simulink model "androidraspberrypisensehat"  (R2025b)
settings: Solver=FixedStepAuto  StartTime=0.0  StopTime=10.0  RelTol=1e-3
libraries: androiduilib x6, androidcommunicationlib x2
settings Model: Creator=The MathWorks, Inc.  LastModifiedBy=The MathWorks, Inc.
settings SolverCC: AlgebraicLoopSolver=TrustRegion  MaxZcPerStep=1.0
settings OptimizationCC: EnhancedBackFolding=on  PassReuseOutputArgsThreshold=0.0  MaxStackSize=64  OptimizeBlockOrder=speed  DifferentSizesBufferReuse=on  OptimizationCustomize=off
settings DebuggingCC: ParameterTunabilityLossMsg=error  UnconnectedInputMsg=warning  UnconnectedOutputMsg=warning  UnconnectedLineMsg=warning
settings HardwareCC: ProdBitPerPointer=32.0  ProdBitPerSizeT=32.0  ProdBitPerPtrDiffT=32.0  ProdLargestAtomicInteger=Long  ProdLargestAtomicFloat=Double  ProdWordSize=32.0  ProdHWDeviceType=ARM Compatible->ARM Cortex-A (32-bit)  UseEmbeddedCoderFeatures=off  UseSimulinkCoderFeatures=off
settings ModelReferenceCC: EnableRefExpFcnMdlSchedulingChecks=on
settings SFSimCC: MATLABDynamicMemAlloc=off
settings RTWCC: SystemTargetFile=ert.tlc  HardwareBoard=Android Device  TLCOptions="-aInlineSetEventsForThisBaseRateFcn=TLC_FALSE -aSuppressMultiTaskScheduler=TLC_FALSE  -aRateBasedStepFcn=0"  TemplateMakefile=ert_default_tmf  GenerateReport=on  RTWVerbose=off  Toolchain=Android SDK/NDK Tools  LaunchReport=on  GPUComputeCapability=3.5  DLArmComputeVersion=19.05  Description=Embedded Coder
settings CodeAppCC: ForceParamTrailComments=on  OperatorAnnotations=on
settings ERTTargetCC: InlinedParameterPlacement=Hierarchical  DynamicArrayContainerType=coder::array  ERTCustomFileBanners=off  SupportContinuousTime=on  SupportNonInlinedSFcns=on  RemoveResetFunc=off  ModelStepFunctionPrototypeControlCompliant=off

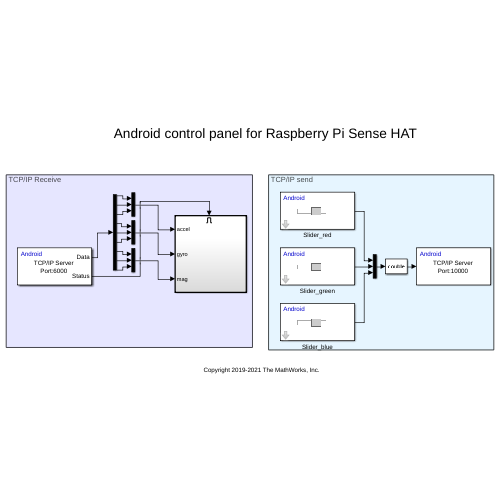
[thumbnail: Simulink's stored preview of the top-level diagram]
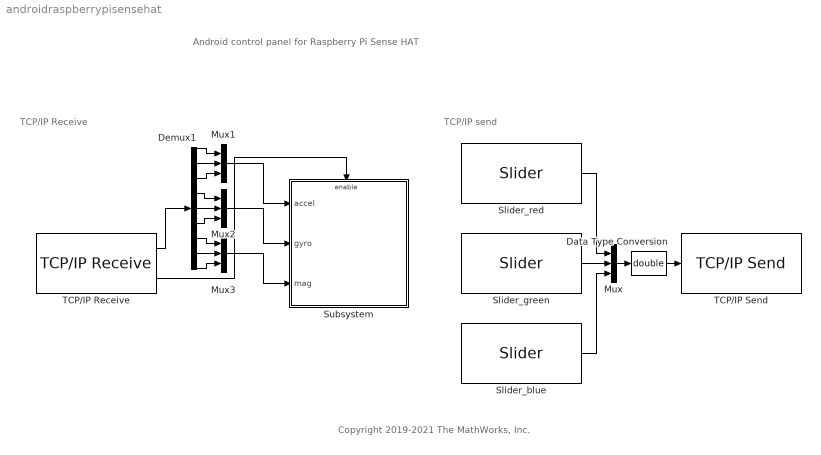
== system androidraspberrypisensehat ==
  note: Android control panel for Raspberry Pi Sense HAT
  note: TCP/IP send
  note: TCP/IP Receive
  note: Copyright 2019-2021 The MathWorks, Inc.
  Data Type Conversion : DataTypeConversion  OutDataTypeStr=double  SaturateOnIntegerOverflow=off  RndMeth=Floor
  Demux1 : Demux  Outputs=9
  Mux{,1..3} (4 alike) : Mux  Inputs=3
  Slider_blue : androiduilib/Slider  Min=1  Value=1  Max=255  Resolution=1  SliderId=androidraspberrypisensehat/Slider_blue  SampleTime=0.5  BlockPlatform=Android
  Slider_green : androiduilib/Slider  Min=1  Value=1  Max=255  Resolution=1  SliderId=androidraspberrypisensehat/Slider_green  SampleTime=0.5  BlockPlatform=Android
  Slider_red : androiduilib/Slider  Min=1  Value=1  Max=255  Resolution=1  SliderId=androidraspberrypisensehat/Slider_red  SampleTime=0.5  BlockPlatform=Android
  Subsystem : Subsystem
  TCP/IP Receive : androidcommunicationlib/TCP//IP Receive  TCPReceiveId=androidraspberrypisensehat/TCP//IP_Receive  Mode_=Server  LocalServerPort_=6000  RemoteAddr_=127.0.0.1  RemoteServerPort_=25000  DataType_=double  DataSize_=9  SampleTime_=0.1  ClientPortBindingSelection_=off  ClientPortToBind_=35000  BlockingMode_=off  BlockTimeout_=0.1
  TCP/IP Send : androidcommunicationlib/TCP//IP Send  TCPSendId=androidraspberrypisensehat/TCP//IP_Send  Mode_=Server  LocalServerPort_=10000  RemoteAddr_=127.0.0.1  RemoteServerPort_=25000  ClientPortBindingSelection_=off  ClientPortToBind_=35000  BlockingMode_=off  BlockTimeout_=0.1
  wires:
  Mux1/1 -> Subsystem/1(accel)
  Mux2/1 -> Subsystem/2(gyro)
  Mux3/1 -> Subsystem/3(mag)
  TCP/IP Receive/2 -> Subsystem/Enable
  Mux/1 -> Data Type Conversion/1
  Slider_red/1 -> Mux/1
  Slider_green/1 -> Mux/2
  Slider_blue/1 -> Mux/3
  TCP/IP Receive/1 -> Demux1/1
  Demux1/2 -> Mux1/2
  Demux1/3 -> Mux1/3
  Demux1/1 -> Mux1/1
  Demux1/5 -> Mux2/2
  Demux1/7 -> Mux3/1
  Demux1/8 -> Mux3/2
  Demux1/9 -> Mux3/3
  Demux1/4 -> Mux2/1
  Demux1/6 -> Mux2/3
  Data Type Conversion/1 -> TCP/IP Send/1

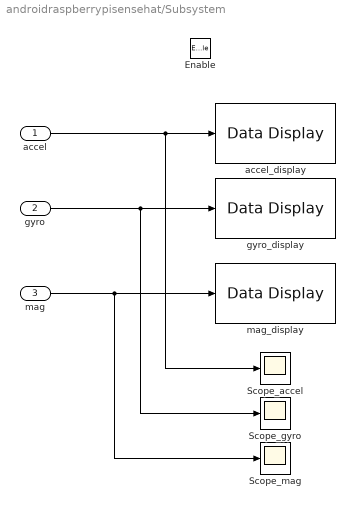
== system androidraspberrypisensehat/Subsystem ==
  accel : Inport
  gyro : Inport  Port=2
  mag : Inport  Port=3
  Enable : EnablePort
  Scope_accel : Scope
  Scope_gyro : Scope
  Scope_mag : Scope
      settings: DataLoggingVariableName=ScopeData2
  accel_display : androiduilib/Data Display  DataDisplayId=androidraspberrypisensehat/Subsystem/accel_display  Format=Float  Precision=6  SimulateUsing=Code generation  blockPlatform=Android
  gyro_display : androiduilib/Data Display  DataDisplayId=androidraspberrypisensehat/Subsystem/gyro_display  Format=Float  Precision=6  SimulateUsing=Code generation  blockPlatform=Android
  "mag_display " : androiduilib/Data Display  DataDisplayId=androidraspberrypisensehat/Subsystem/mag_display_  Format=Float  Precision=6  SimulateUsing=Code generation  blockPlatform=Android
  wires:
  gyro/1 -> Scope_gyro/1, gyro_display/1
  mag/1 -> Scope_mag/1, "mag_display "/1
  accel/1 -> Scope_accel/1, accel_display/1
